simulink model "asmc_edward"  (R2022a)
settings: Solver=FixedStepAuto  StartTime=0.0  StopTime=10  FixedStep=0.001  RelTol=1e-3
undefined symbols (not defined in the file or in its folder): r0
settings Model: Creator=randolf  LastModifiedBy=randolf

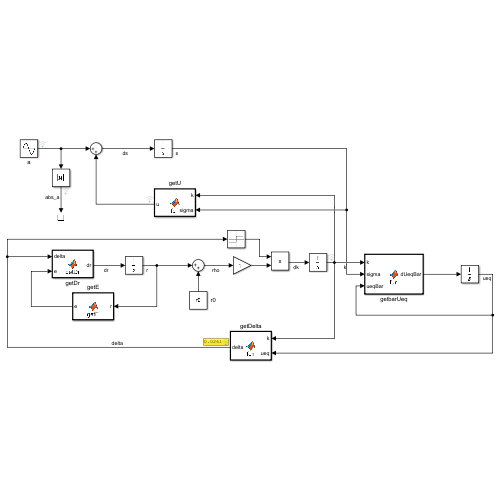
[thumbnail: Simulink's stored preview of the top-level diagram]
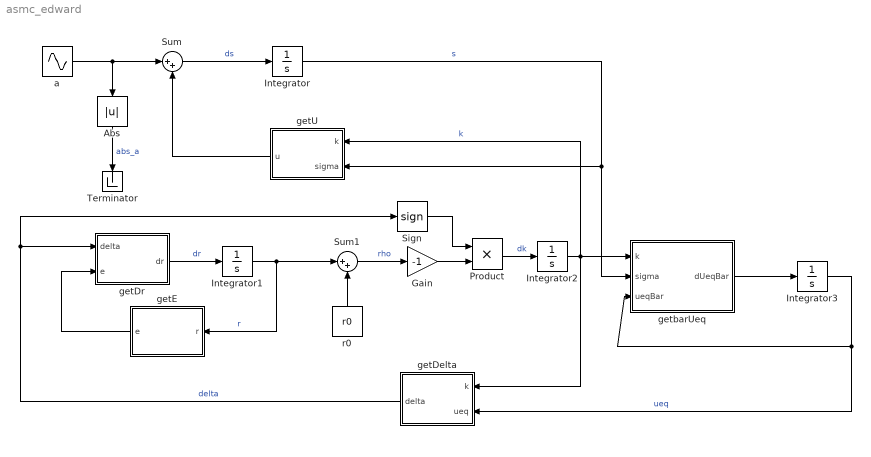
== system asmc_edward ==
  Abs : Abs  SaturateOnIntegerOverflow=off
  Gain : Gain  Gain=-1
  Integrator{,1..3} (4 alike) : Integrator
  Product : Product
  Sign : Signum
  Sum : Sum  Inputs=|++
  Sum1 : Sum  Inputs=|++
  Terminator : Terminator
  a : Sin  SampleTime=0
  getDelta : MATLAB Function  TreatAsAtomicUnit=on
  getDr : MATLAB Function  TreatAsAtomicUnit=on
  getE : MATLAB Function  TreatAsAtomicUnit=on
  getU : MATLAB Function  TreatAsAtomicUnit=on
  getbarUeq : MATLAB Function  TreatAsAtomicUnit=on
  r0 : Constant  Value=r0
  wires:
  a/1 -> Abs/1, Sum/1
  Sum/1 -> Integrator/1  "ds"
  Integrator/1 -> getbarUeq/2(sigma), getU/2(sigma)  "s"
  getDr/1(dr) -> Integrator1/1  "dr"
  Integrator1/1 -> Sum1/1, getE/1(r)  "r"
  getE/1(e) -> getDr/2(e)
  Sum1/1 -> Gain/1  "rho"
  Gain/1 -> Product/2
  Sign/1 -> Product/1
  Product/1 -> Integrator2/1  "dk"
  Integrator2/1 -> getU/1(k), getDelta/1(k), getbarUeq/1(k)  "k"
  getbarUeq/1(dUeqBar) -> Integrator3/1
  Integrator3/1 -> getDelta/2(ueq), getbarUeq/3(ueqBar)  "ueq"
  getDelta/1(delta) -> Sign/1, getDr/1(delta)  "delta"
  r0/1 -> Sum1/2
  getU/1(u) -> Sum/2
  Abs/1 -> Terminator/1  "abs_a"

== matlab function asmc_edward/getDr ==
  data: delta input; dr output size=1; e input
function dr = getDr(delta, e)
    coder.extrinsic('evalin');
    gamma = 0.0;
    r0 = 0.0;
    
    gamma = evalin('base','gamma');
    r0 = evalin("base", 'r0');

    dr = gamma*abs(delta) + r0*sqrt(gamma)*sign(e);
end

== matlab function asmc_edward/getbarUeq ==
  data: k input; dUeqBar output size=1; sigma input; ueqBar input
function dUeqBar = fun(k, sigma, ueqBar)
    coder.extrinsic('evalin');
    eta = 0.0;
    tau = 0.0;
    eta = evalin('base','eta');
    tau = evalin('base','tau');
    dUeqBar = 1/tau*(-(k+eta)*sign(sigma)-ueqBar);
end

== matlab function asmc_edward/getDelta ==
  data: k input; delta output size=1; ueq input
function delta = fcn(k, ueq)
    coder.extrinsic('evalin');
    alp = 0.0;
    epsilon = 0.0;
    
    alp = evalin('base','alp');
    epsilon = evalin('base','epsilon');
    delta = k - 1/alp*abs(ueq)-epsilon;
end

== matlab function asmc_edward/getU ==
  data: k input; u output size=1; sigma input
function u = fcn(k, sigma)
    coder.extrinsic('evalin');

    eta = 0.0;
    
    eta = evalin("base", 'eta');

    u = -(k+eta)*sign(sigma);
end

== matlab function asmc_edward/getE ==
  data: r input; e output size=1
function e = getE(r)
   coder.extrinsic('evalin');

   q = 0.0;
   alp = 0.0;
   a1 = 0.0;
   
   q = evalin('base','q');
   alp = evalin('base','alp');
   a1 = evalin('base','a1');
   e =  (q*a1)/alp - r;
end
